simulink model "simdyn"  (R2014a)
settings: Solver=ode45  StartTime=0.0  StopTime=10.0  RelTol=1e-3
PreLoadFcn:
  | if(~any(strcmp(who,'Testumgebung')))
  | 
  | L1 = link([0 4 0 0]);
  | L2 = link([0 3 0 0]);
  | L3 = link([0 2 0 0]);
  | 
  | L1.m = 20;
  | L2.m = 15;
  | L3.m = 10;
  | 
  | L1.r = [-2 0 0]';
  | L2.r = [-1.5 0 0]';
  | L3.r = [-1 0 0]';
  | 
  | L1.I = [0 0 0; 0 0 0; 0 0 0.5];
  | L2.I = [0 0 0; 0 0 0; 0 0 0.2];
  | L3.I = [0 0 0; 0 0 0; 0 0 0.1];
  | 
  | L1.Jm = 0;
  | L2.Jm = 0;
  | L3.Jm = 0;
  | 
  | L1.G = 1;
  | L2.G = 1;
  | L3.G = 1;
  | 
  | Rob = robot({L1 L2 L3}, 'Rob');
  | 
  | Rob.gravity = [0 9.81 0]';
  | 
  | clear('L1','L2','L3')
  | end
settings Model: Creator=user  LastModifiedBy=Wolfgang
settings SolverCC: ZeroCrossAlgorithm=Adaptive
settings OptimizationCC: SimCompilerOptimization=On
settings DebuggingCC: UnderspecifiedInitializationDetection=Classic  SolverPrmCheckMsg=none

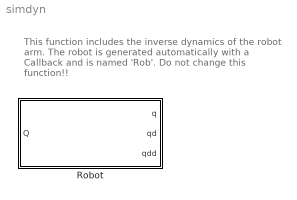
== system simdyn ==
  note: This function includes the inverse dynamics
      | of the robot arm. The robot is generated
      | automatically with a Callback and is named 'Rob'.
      | Do not change this function!!
  Robot : Subsystem  InitFcn=|  mask{robot=Rob, q0=[0 0 0]}
      | set_param(gcb,'q0','[0 0 0]');
      | 
      | if(~any(strcmp(who,'Testumgebung')))
      | warning off Simulink:Engine:OutputNotConnected
      | 
      | L1 = Link([0 0 4 0]);
      | L2 = Link([0 0 3 0]);
      | L3 = Link([0 0 2 0]);
      | 
      | L1.m = 20;
      | L2.m = 15;
      | L3.m = 10;
      | 
      | L1.r = [-2 0 0]';
      | L2.r = [-1.5 0 0]';
      | L3.r = [-1 0 0]';
      | 
      | L1.I = [0 0 0; 0 0 0; 0 0 0.5];
      | L2.I = [0 0 0; 0 0 0; 0 0 0.2];
      | L3.I = [0 0 0; 0 0 0; 0 0 0.1];
      | 
      | L1.Jm = 0;
      | L2.Jm = 0;
      | L3.Jm = 0;
      | 
      | L1.G = 1;
      | L2.G = 1;
      | L3.G = 1;
      | 
      | Rob = SerialLink([L1 L2 L3],'name', 'Rob');
      | 
      | Rob.gravity = [0 9.81 0]';
      | 
      | clear('L1','L2','L3')
      | 
      | if(~strcmp(get_param(gcb,'Robot'),'Rob'))
      | set_param(gcb,'Robot','Rob');
      | warning('Verändern sie nicht den Namen des Roboters. Ein Roboter mit dem Namen "Rob" wird automatisch in einer Callback Funktion erzeugt.')
      | end
      | end
      mask prompts: robot "Robot object"; q0 "Initial state"
      mask help: Rigid-body dynamic model of robot.
      mask init:
      | n = robot.n;
      | name = robot.name;
      mask Help: Simulates the forward (direct) rigid-body dynamics of the robot described by the given robot object.
      mask Display:
      | port_label('input', 1, 'tau')
      | port_label('output', 1, 'q')
      | port_label('output', 2, 'qd')
      | port_label('output', 3, 'qdd')
      | text(0.1, 0.9,  robot.name, 'horizontalAlignment', 'left')

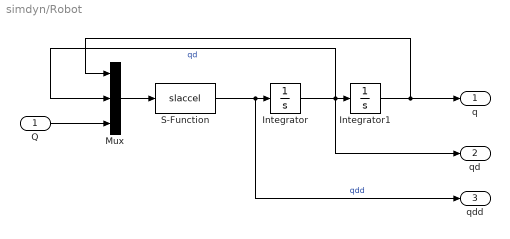
== system simdyn/Robot ==
  Q : Inport
  Integrator : Integrator
  Integrator1 : Integrator  InitialCondition=q0
  Mux : Mux  Inputs=3
  S-Function : S-Function  FunctionName=slaccel  Parameters=robot  EnableBusSupport=off
  q : Outport
  qd : Outport  Port=2
  qdd : Outport  Port=3
  wires:
  Mux/1 -> S-Function/1
  S-Function/1 -> qdd/1, Integrator/1  "qdd"
  Integrator/1 -> qd/1, Integrator1/1, Mux/2  "qd"
  Q/1 -> Mux/3
  Integrator1/1 -> q/1, Mux/1
